simulink model "system_model"  (R2022b)
settings: Solver=VariableStepAuto  StartTime=0.0  StopTime=10  RelTol=1e-3
values from neighbouring files (symbols this model uses):
  A = [0      0      0      1      0      0 ... (first row only)    [load_parameter.m]    (also in parameter.m)
  B = [0      0 ... (first row only)    [load_parameter.m]    (also in parameter.m)
  C = [1   0   0   0   0   0 ... (first row only)    [load_parameter.m]    (also in parameter.m)
  C2 = [1 0 0 0 0 0; 0 0 1 0 0 0]    [main.m]
  K11 = place(A,B,p)    [pole_placement.m]
  K2 = lqr_control(A, B)    [main.m]    (also in servo.m = K(:,7:9))
  x0 = [0.2;  -0.1;   0.15;  -1;  0.8;   0]    [load_parameter.m]    (also in parameter.m)
undefined symbols (not defined in the file or in its folder): F4, K4
settings Model: Creator=cyh  LastModifiedBy=cyh
settings DataIOCC: InitialState=x0

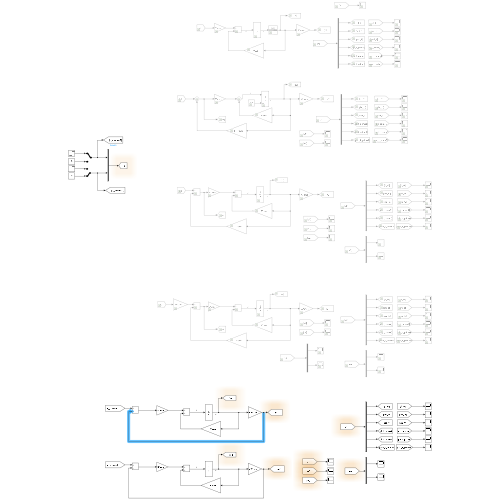
[thumbnail: Simulink's stored preview of the top-level diagram]
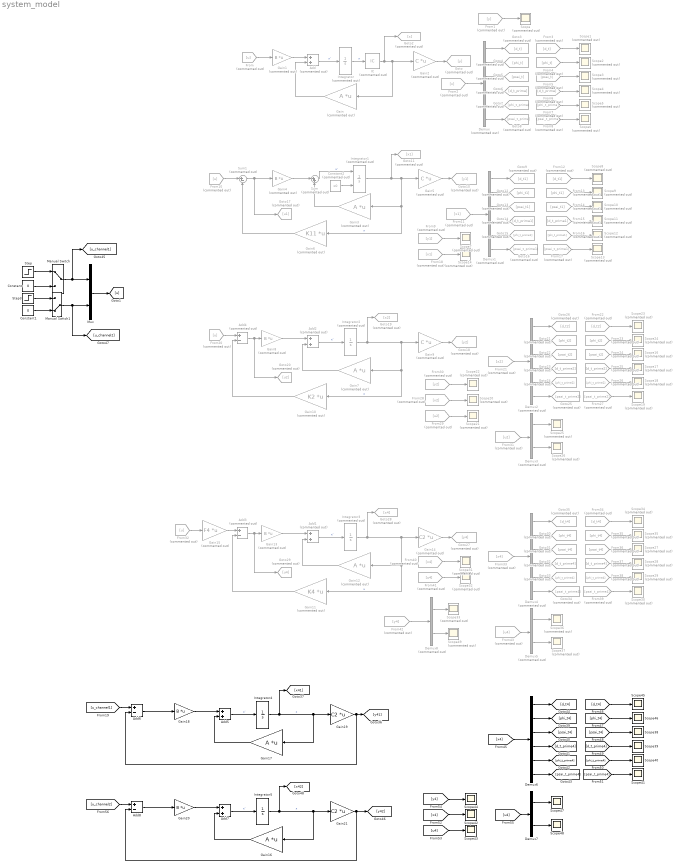
== system system_model ==
  Add : Sum  Commented=on
  Add1 : Sum  Commented=on
  Add2 : Sum  Commented=on
  Add3 : Sum  Commented=on  Inputs=+-
  Add4 : Sum  Commented=on  Inputs=+-
  Add5 : Sum
  Add6 : Sum  Inputs=+-
  Add7 : Sum
  Add8 : Sum  Inputs=+-
  Constant : Constant  Value=0
  Constant1 : Constant  Value=0
  Constant2 : Constant  Commented=on  Value=x0
  Demux{,1..2,4} (4 alike) : Demux  Commented=on  Outputs=6
  Demux3 : Demux  Commented=on  Outputs=2
  Demux5 : Demux  Commented=on  Outputs=2
  Demux6 : Demux  Outputs=6
  Demux7 : Demux  Outputs=2
  Demux8 : Demux  Commented=on  Outputs=2
  From{,10,20,32} (4 alike) : From  Commented=on  GotoTag=u
  From1 : From  Commented=on  GotoTag=y
  From11 : From  Commented=on  GotoTag=x1
  From12 : From  Commented=on  GotoTag=d_t1
  From13 : From  Commented=on  GotoTag=phi_t1
  From14 : From  Commented=on  GotoTag=psai_t1
  From15 : From  Commented=on  GotoTag=d_t_prime1
  From16 : From  Commented=on  GotoTag=phi_t_prime1
  From17 : From  Commented=on  GotoTag=psai_t_prime1
  From18 : From  Commented=on  GotoTag=x1
  From2 : From  Commented=on  GotoTag=x
  From21 : From  Commented=on  GotoTag=x2
  From22 : From  Commented=on  GotoTag=d_t2
  From23 : From  Commented=on  GotoTag=phi_t2
  From24 : From  Commented=on  GotoTag=psai_t2
  From25 : From  Commented=on  GotoTag=d_t_prime2
  From26 : From  Commented=on  GotoTag=phi_t_prime2
  From27 : From  Commented=on  GotoTag=psai_t_prime2
  From28 : From  Commented=on  GotoTag=x2
  From29 : From  Commented=on  GotoTag=u2
  From3 : From  Commented=on  GotoTag=d_t
  From30 : From  Commented=on  GotoTag=y2
  From31 : From  Commented=on  GotoTag=u2
  From33 : From  Commented=on  GotoTag=x4
  From34 : From  Commented=on  GotoTag=d_t4
  From35 : From  Commented=on  GotoTag=phi_t4
  From36 : From  Commented=on  GotoTag=psai_t4
  From37 : From  Commented=on  GotoTag=d_t_prime4
  From38 : From  Commented=on  GotoTag=phi_t_prime4
  From39 : From  Commented=on  GotoTag=psai_t_prime4
  From4 : From  Commented=on  GotoTag=phi_t
  From40 : From  Commented=on  GotoTag=x4
  From41 : From  Commented=on  GotoTag=u4
  From42 : From  Commented=on  GotoTag=y4
  From43 : From  Commented=on  GotoTag=u4
  From5 : From  Commented=on  GotoTag=psai_t
  From6 : From  Commented=on  GotoTag=d_t_prime
  From7 : From  Commented=on  GotoTag=phi_t_prime
  From8 : From  Commented=on  GotoTag=psai_t_prime
  From9 : From  Commented=on  GotoTag=y1
  Gain{,3,7,12} (4 alike) : Gain  Commented=on  Gain=A  Multiplication=Matrix(K*u) (u vector)
  Gain{1,4,8,13} (4 alike) : Gain  Commented=on  Gain=B  Multiplication=Matrix(K*u) (u vector)
  Gain10 : Gain  Commented=on  Gain=K2  Multiplication=Matrix(K*u) (u vector)
  Gain11 : Gain  Commented=on  Gain=K4  Multiplication=Matrix(K*u) (u vector)
  Gain14 : Gain  Commented=on  Gain=C2  Multiplication=Matrix(K*u) (u vector)
  Gain15 : Gain  Commented=on  Gain=F4  Multiplication=Matrix(K*u) (u vector)
  Gain16 : Gain  Gain=A  Multiplication=Matrix(K*u) (u vector)
  Gain17 : Gain  Gain=A  Multiplication=Matrix(K*u) (u vector)
  Gain18 : Gain  Gain=B  Multiplication=Matrix(K*u) (u vector)
  Gain19 : Gain  Gain=C2  Multiplication=Matrix(K*u) (u vector)
  Gain2 : Gain  Commented=on  Gain=C  Multiplication=Matrix(K*u) (u vector)
  Gain20 : Gain  Gain=B  Multiplication=Matrix(K*u) (u vector)
  Gain21 : Gain  Gain=C2  Multiplication=Matrix(K*u) (u vector)
  Gain5 : Gain  Commented=on  Gain=C  Multiplication=Matrix(K*u) (u vector)
  Gain6 : Gain  Commented=on  Gain=K11  Multiplication=Matrix(K*u) (u vector)
  Gain9 : Gain  Commented=on  Gain=C  Multiplication=Matrix(K*u) (u vector)
  Goto : Goto  Commented=on  GotoTag=y
  Goto10 : Goto  Commented=on  GotoTag=y1
  Goto11 : Goto  Commented=on  GotoTag=x1
  Goto12 : Goto  Commented=on  GotoTag=phi_t1
  Goto13 : Goto  Commented=on  GotoTag=psai_t1
  Goto14 : Goto  Commented=on  GotoTag=d_t_prime1
  Goto15 : Goto  Commented=on  GotoTag=phi_t_prime1
  Goto16 : Goto  Commented=on  GotoTag=psai_t_prime1
  Goto17 : Goto  Commented=on  GotoTag=u1
  Goto18 : Goto  Commented=on  GotoTag=y2
  Goto19 : Goto  Commented=on  GotoTag=x2
  Goto2 : Goto  Commented=on  GotoTag=x
  Goto20 : Goto  Commented=on  GotoTag=u2
  Goto21 : Goto  Commented=on  GotoTag=phi_t2
  Goto22 : Goto  Commented=on  GotoTag=psai_t2
  Goto23 : Goto  Commented=on  GotoTag=d_t_prime2
  Goto24 : Goto  Commented=on  GotoTag=phi_t_prime2
  Goto25 : Goto  Commented=on  GotoTag=psai_t_prime2
  Goto26 : Goto  Commented=on  GotoTag=d_t2
  Goto27 : Goto  Commented=on  GotoTag=y4
  Goto28 : Goto  Commented=on  GotoTag=x4
  Goto29 : Goto  Commented=on  GotoTag=u4
  Goto3 : Goto  Commented=on  GotoTag=d_t
  Goto30 : Goto  Commented=on  GotoTag=phi_t4
  Goto31 : Goto  Commented=on  GotoTag=psai_t4
  Goto32 : Goto  Commented=on  GotoTag=d_t_prime4
  Goto33 : Goto  Commented=on  GotoTag=phi_t_prime4
  Goto34 : Goto  Commented=on  GotoTag=psai_t_prime4
  Goto35 : Goto  Commented=on  GotoTag=d_t4
  Goto4 : Goto  Commented=on  GotoTag=phi_t
  Goto5 : Goto  Commented=on  GotoTag=psai_t
  Goto6 : Goto  Commented=on  GotoTag=d_t_prime
  Goto7 : Goto  Commented=on  GotoTag=phi_t_prime
  Goto8 : Goto  Commented=on  GotoTag=psai_t_prime
  Goto9 : Goto  Commented=on  GotoTag=d_t1
  IC : InitialCondition  Commented=on  Value=x0
  Integrator : Integrator  Commented=on
  Integrator1 : Integrator  Commented=on  InitialConditionSource=external  InitialCondition=x0
  Integrator2 : Integrator  Commented=on  InitialCondition=x0
  Integrator3 : Integrator  Commented=on  InitialCondition=x0
  Integrator4 : Integrator  InitialCondition=x0
  Integrator5 : Integrator  InitialCondition=x0
  Manual Switch : ManualSwitch
  Manual Switch1 : ManualSwitch  CurrentSetting=0
  Mux : Mux  Inputs=2
  Scope{,1..14,16..37,49} (38 alike) : Scope  Commented=on
  Scope{38..48} (11 alike) : Scope
  Step : Step  Time=0  SampleTime=0
  Step3 : Step  Time=0  SampleTime=0
  Sum : Sum  Commented=on  Inputs=|++
  Sum1 : Sum  Commented=on  Inputs=|+-
  wires:
  Integrator/1 -> IC/1  "x"
  Add/1 -> Integrator/1  "x'"
  Gain/1 -> Add/2
  Gain1/1 -> Add/1
  From/1 -> Gain1/1
  IC/1 -> Goto2/1, Gain2/1, Gain/1
  Gain2/1 -> Goto/1
  Mux/1 -> [u]
  From1/1 -> Scope/1
  From2/1 -> Demux/1
  Demux/1 -> Goto3/1
  Demux/2 -> Goto4/1
  Demux/3 -> Goto5/1
  Demux/4 -> Goto6/1
  From3/1 -> Scope1/1
  From4/1 -> Scope2/1
  From5/1 -> Scope3/1
  From6/1 -> Scope4/1
  From7/1 -> Scope5/1
  From8/1 -> Scope6/1
  Integrator1/1 -> Goto11/1, Gain6/1, Gain3/1, Gain5/1  "x"
  Gain5/1 -> Goto10/1
  From16/1 -> Scope12/1
  From12/1 -> Scope8/1
  Demux1/2 -> Goto12/1
  From14/1 -> Scope10/1
  Demux1/3 -> Goto13/1
  From15/1 -> Scope11/1
  Demux1/4 -> Goto14/1
  From9/1 -> Scope7/1
  From17/1 -> Scope13/1
  From13/1 -> Scope9/1
  Demux1/1 -> Goto9/1
  From11/1 -> Demux1/1
  Sum/1 -> Integrator1/1  "x'"
  Sum1/1 -> Goto17/1, Gain4/1
  Step/1 -> Manual Switch/1
  Constant1/1 -> Manual Switch1/2
  Constant/1 -> Manual Switch/2
  Step3/1 -> Manual Switch1/1
  From18/1 -> Scope14/1
  Gain8/1 -> Add2/1
  Add2/1 -> Integrator2/1  "x'"
  Gain7/1 -> Add2/2
  Add4/1 -> Goto20/1, Gain8/1
  From20/1 -> Add4/1
  Gain9/1 -> Goto18/1
  Integrator2/1 -> Gain10/1, Gain7/1, Gain9/1, Goto19/1  "x"
  Gain10/1 -> Add4/2
  Demux2/4 -> Goto23/1
  From21/1 -> Demux2/1
  Demux2/2 -> Goto21/1
  Demux2/1 -> Goto26/1
  From27/1 -> Scope19/1
  From22/1 -> Scope23/1
  Demux2/3 -> Goto22/1
  From24/1 -> Scope16/1
  From26/1 -> Scope18/1
  From25/1 -> Scope17/1
  From23/1 -> Scope24/1
  From30/1 -> Scope22/1
  From29/1 -> Scope21/1
  From28/1 -> Scope20/1
  Manual Switch1/1 -> [u_channel2], Mux/2
  Manual Switch/1 -> [u_channel1], Mux/1
  Demux/5 -> Goto7/1
  Demux/6 -> Goto8/1
  Demux1/5 -> Goto15/1
  Demux1/6 -> Goto16/1
  Demux2/5 -> Goto24/1
  Demux2/6 -> Goto25/1
  Gain4/1 -> Sum/1
  Gain3/1 -> Sum/2
  From10/1 -> Sum1/1
  Gain6/1 -> Sum1/2
  Constant2/1 -> Integrator1/2
  From31/1 -> Demux3/1
  Demux3/1 -> Scope25/1
  Demux3/2 -> Scope26/1
  From34/1 -> Scope34/1
  Gain11/1 -> Add3/2
  Add3/1 -> Goto29/1, Gain13/1
  Demux4/4 -> Goto32/1
  From39/1 -> Scope30/1
  Demux5/2 -> Scope37/1
  Demux4/1 -> Goto35/1
  Gain12/1 -> Add1/2
  Integrator3/1 -> Gain11/1, Gain12/1, Gain14/1, Goto28/1  "x"
  Gain14/1 -> Goto27/1
  From35/1 -> Scope35/1
  From37/1 -> Scope28/1
  From36/1 -> Scope27/1
  Demux4/2 -> Goto30/1
  From33/1 -> Demux4/1
  Gain13/1 -> Add1/1
  From40/1 -> Scope31/1
  From43/1 -> Demux5/1
  Add1/1 -> Integrator3/1  "x'"
  From38/1 -> Scope29/1
  From41/1 -> Scope32/1
  Demux4/5 -> Goto33/1
  Demux4/3 -> Goto31/1
  Demux5/1 -> Scope36/1
  Demux4/6 -> Goto34/1
  Gain15/1 -> Add3/1
  From32/1 -> Gain15/1
  [phi_t_prime4] -> Scope40/1
  Integrator4/1 -> Gain17/1, Gain19/1, [x41]  "x"
  Demux7/1 -> Scope47/1
  [u4] -> Scope43/1
  [u4] -> Demux7/1
  [d_t4] -> Scope45/1
  Gain18/1 -> Add5/1
  Demux6/2 -> [phi_t4]
  Demux6/4 -> [d_t_prime4]
  [psai_t4] -> Scope38/1
  [psai_t_prime4] -> Scope41/1
  Demux6/6 -> [psai_t_prime4]
  Demux6/1 -> [d_t4]
  Demux6/3 -> [psai_t4]
  [y4] -> Scope44/1
  Gain17/1 -> Add5/2
  [phi_t4] -> Scope46/1
  Demux7/2 -> Scope48/1
  Demux6/5 -> [phi_t_prime4]
  [d_t_prime4] -> Scope39/1
  Add5/1 -> Integrator4/1  "x'"
  [u_channel1] -> Add6/1
  [x4] -> Demux6/1
  [x4] -> Scope42/1
  Gain19/1 -> Add6/2, [y41]
  From42/1 -> Demux8/1
  Demux8/1 -> Scope33/1
  Demux8/2 -> Scope49/1
  Add6/1 -> Gain18/1
  Gain21/1 -> Add8/2, [y42]
  Gain16/1 -> Add7/2
  Gain20/1 -> Add7/1
  [u_channel2] -> Add8/1
  Add8/1 -> Gain20/1
  Integrator5/1 -> Gain16/1, Gain21/1, [x42]  "x"
  Add7/1 -> Integrator5/1  "x'"
